simulink model "modern02"  (R2016b)
settings: Solver=VariableStepAuto  StartTime=0.0  StopTime=20  RelTol=1e-3
settings Model: Creator=user  LastModifiedBy=user

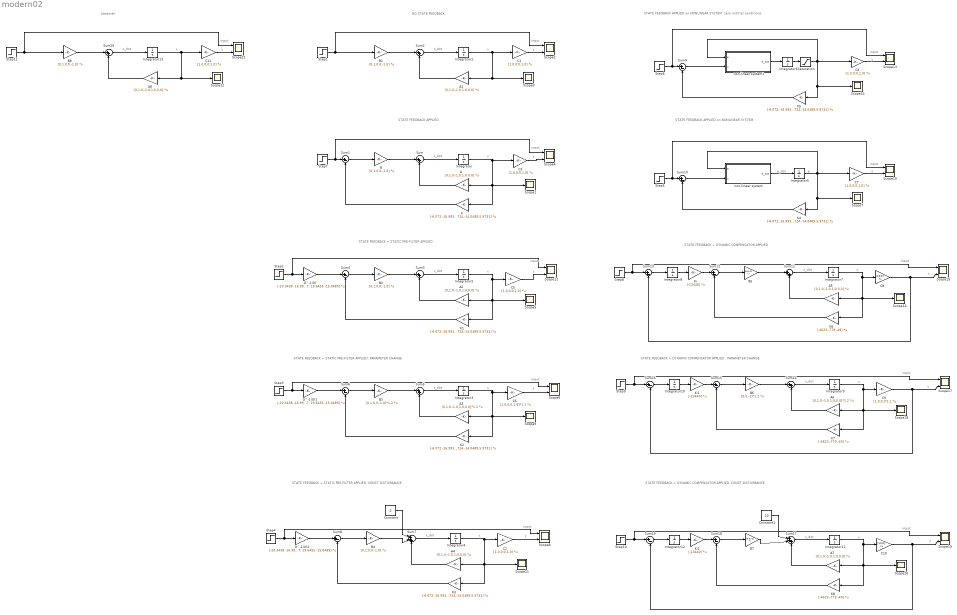
== system modern02 ==
  note: e_dot
  note: e
  note: y
  note: STATE FEEDBACK APPLIED
  note: NO STATE FEEDBACK
  note: input
  note: y
  note: x
  note: x_dot
  note: input
  note: y
  note: x
  note: x_dot
  note: STATE FEEDBACK + STATIC PRE-FILTER APPLIED
  note: input
  note: y
  note: x
  note: x_dot
  note: STATE FEEDBACK + STATIC PRE-FILTER APPLIED: PARAMETER CHANGE
  note: input
  note: y
  note: x
  note: x_dot
  note: STATE FEEDBACK + STATIC PRE-FILTER APPLIED: CONST DISTURBANCE
  note: input
  note: y
  note: x
  note: x_dot
  note: STATE FEEDBACK APPLIED on NONLINEAR SYSTEM
  note: input
  note: y
  note: STATE FEEDBACK APPLIED on NONLINEAR SYSTEM: zero inititial conditions
  note: input
  note: y
  note: STATE FEEDBACK + DYNAMIC COMPENSATOR APPLIED
  note: input
  note: x
  note: x_dot
  note: y
  note: STATE FEEDBACK + DYNAMIC COMPENSATOR APPLIED : PARAMETER CHANGE
  note: input
  note: x
  note: x_dot
  note: STATE FEEDBACK + DYNAMIC COMPENSATOR APPLIED: CONST DISTURBANCE
  note: y
  note: input
  note: x
  note: x_dot
  note: observer
  note: input
  note: y
  note: x
  note: x_dot
  A{,1..2,4..5,7..8} (7 alike) : Gain  Gain=[0,1,0;-1,0,1;0,0,0]  Multiplication=Matrix(K*u)
  A3 : Gain  Gain=[0,1,0;-1,0,1;0,0,0]*1.1  Multiplication=Matrix(K*u)
  A6 : Gain  Gain=[0,1,0;-1,0,1;0,0,0]*1.2  Multiplication=Matrix(K*u)
  B{,1..2,4,8} (5 alike) : Gain  Gain=[0,1;0,0;-1,0]  Multiplication=Matrix(K*u)
  B3 : Gain  Gain=[0,1;0,0;-1,0]*1.2  Multiplication=Matrix(K*u)
  B5 : Gain  Gain=[0;0;-1]  Multiplication=Matrix(K*u)
  B6 : Gain  Gain=[0;0;-1]*1.2  Multiplication=Matrix(K*u)
  B7 : Gain  Gain=[0;0;-1]  Multiplication=Matrix(K*u)
  C{1..5,7,11} (7 alike) : Gain  Gain=[1,0,0;0,1,0]  Multiplication=Matrix(K*u)
  C10 : Gain  Gain=[1,0,0;]  Multiplication=Matrix(K*u)
  C6 : Gain  Gain=[1,0,0;0,1,0]*1.1  Multiplication=Matrix(K*u)
  C8 : Gain  Gain=[1,0,0;]  Multiplication=Matrix(K*u)
  C9 : Gain  Gain=[1,0,0;]*1.1  Multiplication=Matrix(K*u)
  Constant : Constant  Value=2
  Constant1 : Constant  Value=10
  G^-1(0) : Gain  Gain=[-20.3438 -16.9937; 19.6455 -15.0489]  Multiplication=Matrix(K*u)
  G^-1(0)1 : Gain  Gain=[-20.3438 -16.9937; 19.6455 -15.0489]  Multiplication=Matrix(K*u)
  G^-1(0)2 : Gain  Gain=[-20.3438 -16.9937; 19.6455 -15.0489]  Multiplication=Matrix(K*u)
  Integrator{,1..4,6..7,9,11,13} (10 alike) : Integrator  InitialCondition=[0,0,0]
  Integrator10 : Integrator  InitialCondition=[0]
  Integrator12 : Integrator  InitialCondition=[0]
  Integrator5 : Integrator  InitialCondition=[-1,-1,-1]
  Integrator8 : Integrator  InitialCondition=[0]
  K{,1..5} (6 alike) : Gain  Gain=[-6.072,-16.9937,-14.3276;13.6724,-14.0489,5.9731]  Multiplication=Matrix(K*u)
  K6 : Gain  Gain=[-4623,-779,-49]  Multiplication=Matrix(K*u)
  K7 : Gain  Gain=[-4623,-779,-49]  Multiplication=Matrix(K*u)
  K8 : Gain  Gain=[-4623,-779,-49]  Multiplication=Matrix(K*u)
  Ki : Gain  Gain=[-13440]  Multiplication=Matrix(K*u)
  Ki1 : Gain  Gain=[-13440]  Multiplication=Matrix(K*u)
  Ki2 : Gain  Gain=[-13440]  Multiplication=Matrix(K*u)
  Saturation : Saturate  UpperLimit=20  LowerLimit=-20
  Scope{1,3,5,7,9,11,14,16,18,20,22} (11 alike) : Scope
  Scope{2,4,6,8,10,12..13,15,17,19,21} (11 alike) : Scope  NumInputPorts=2
  Step{1..7,11} (8 alike) : Step  Time=[2,4]  Before=[0,0]  After=[1,-.3]  SampleTime=0
  Step10 : Step  Time=[2]  Before=[0]  After=[1]  SampleTime=0
  Step8 : Step  Time=[2]  Before=[0]  After=[1]  SampleTime=0
  Step9 : Step  Time=[2]  Before=[0]  After=[1]  SampleTime=0
  Sum{,2..3,5,11,14,20} (7 alike) : Sum  Inputs=|++
  Sum{1,4,6,8..10,12..13,15..16,18..19} (12 alike) : Sum  Inputs=|+-
  Sum17 : Sum  Inputs=|+++
  Sum7 : Sum  Inputs=|+++
  non-linear system : MATLAB Function  TreatAsAtomicUnit=on
  non-linear system1 : MATLAB Function  TreatAsAtomicUnit=on
  wires:
  Sum/1 -> Integrator/1
  Integrator/1 -> C3/1, Scope1/1, K/1, A/1
  B/1 -> Sum/1
  A/1 -> Sum/2
  Sum1/1 -> B/1
  K/1 -> Sum1/2
  Step7/1 -> Scope4/1, Sum1/1
  Sum2/1 -> Integrator1/1
  Integrator1/1 -> Scope3/1, A1/1, C1/1
  B1/1 -> Sum2/1
  A1/1 -> Sum2/2
  Step1/1 -> B1/1, Scope2/1
  C1/1 -> Scope2/2
  Sum3/1 -> Integrator2/1
  Integrator2/1 -> C5/1, Scope5/1, K1/1, A2/1
  B2/1 -> Sum3/1
  A2/1 -> Sum3/2
  Sum4/1 -> B2/1
  K1/1 -> Sum4/2
  Step2/1 -> Scope12/1, G^-1(0)/1
  G^-1(0)/1 -> Sum4/1
  Sum5/1 -> Integrator3/1
  Integrator3/1 -> C6/1, Scope9/1, K2/1, A3/1
  B3/1 -> Sum5/1
  A3/1 -> Sum5/2
  Sum6/1 -> B3/1
  K2/1 -> Sum6/2
  C6/1 -> Scope6/2
  Step3/1 -> G^-1(0)1/1, Scope6/1
  G^-1(0)1/1 -> Sum6/1
  Sum7/1 -> Integrator4/1
  Integrator4/1 -> C2/1, Scope11/1, K3/1, A4/1
  B4/1 -> Sum7/2
  A4/1 -> Sum7/3
  Sum8/1 -> B4/1
  K3/1 -> Sum8/2
  C2/1 -> Scope8/2
  Step4/1 -> Scope8/1, G^-1(0)2/1
  G^-1(0)2/1 -> Sum8/1
  Constant/1 -> Sum7/1
  non-linear system/1(e_dot) -> Integrator5/1
  K4/1 -> Sum10/2
  Step5/1 -> Scope10/1, Sum10/1
  C7/1 -> Scope10/2
  Integrator5/1 -> C7/1, Scope7/1, K4/1, non-linear system/1(e)
  Sum10/1 -> non-linear system/2(u)
  C3/1 -> Scope4/2
  C5/1 -> Scope12/2
  non-linear system1/1(e_dot) -> Integrator6/1
  K5/1 -> Sum9/2
  Step6/1 -> Scope13/1, Sum9/1
  C4/1 -> Scope13/2
  Integrator6/1 -> Saturation/1
  Sum9/1 -> non-linear system1/2(u)
  Saturation/1 -> C4/1, Scope14/1, K5/1, non-linear system1/1(e)
  Sum11/1 -> Integrator7/1
  Integrator7/1 -> C8/1, Scope16/1, K6/1, A5/1
  B5/1 -> Sum11/1
  A5/1 -> Sum11/2
  Sum12/1 -> B5/1
  K6/1 -> Sum12/2
  Step8/1 -> Sum13/1, Scope15/1
  Ki/1 -> Sum12/1
  C8/1 -> Sum13/2, Scope15/2
  Integrator8/1 -> Ki/1
  Sum13/1 -> Integrator8/1
  Sum14/1 -> Integrator9/1
  Integrator9/1 -> C9/1, Scope18/1, K7/1, A6/1
  B6/1 -> Sum14/1
  A6/1 -> Sum14/2
  Sum15/1 -> B6/1
  K7/1 -> Sum15/2
  Step9/1 -> Sum16/1, Scope17/1
  Ki1/1 -> Sum15/1
  C9/1 -> Sum16/2, Scope17/2
  Integrator10/1 -> Ki1/1
  Sum16/1 -> Integrator10/1
  Sum17/1 -> Integrator11/1
  Integrator11/1 -> C10/1, Scope20/1, K8/1, A7/1
  B7/1 -> Sum17/2
  A7/1 -> Sum17/3
  Sum18/1 -> B7/1
  K8/1 -> Sum18/2
  Step10/1 -> Sum19/1, Scope19/1
  Ki2/1 -> Sum18/1
  C10/1 -> Sum19/2, Scope19/2
  Integrator12/1 -> Ki2/1
  Sum19/1 -> Integrator12/1
  Constant1/1 -> Sum17/1
  Sum20/1 -> Integrator13/1
  Integrator13/1 -> Scope22/1, A8/1, C11/1
  B8/1 -> Sum20/1
  A8/1 -> Sum20/2
  Step11/1 -> B8/1, Scope21/1
  C11/1 -> Scope21/2

== matlab function modern02/non-linear system1 ==
  data: e input; e_dot output; u input
function e_dot  = fcn(e,u)
e_dot = [0;0;0];
e_dot(1)=(1-u(1))*e(2) + cos(e(3))+(u(2)-1);
e_dot(2)=(u(1)-1)*e(2) + sin(e(1));
e_dot(3)=-u(1);

== matlab function modern02/non-linear system ==
  data: e input; e_dot output; u input
function e_dot  = fcn(e,u)
e_dot = [0;0;0];
e_dot(1)=(1-u(1))*e(2) + cos(e(3))+(u(2)-1);
e_dot(2)=(u(1)-1)*e(2) + sin(e(1));
e_dot(3)=-u(1);
